simulink model "model_discrete"  (R2021b)
settings: Solver=FixedStepAuto  StartTime=0.0  StopTime=StopTime  FixedStep=T  RelTol=1e-3  EnableMultiTasking=on
undefined symbols (not defined in the file): K_disc, Knorm_disc, mtrxA_disc, mtrxB_disc, mtrxC_disc, Out, T
settings Model: Creator=vkad  LastModifiedBy=vkad
settings DataIOCC: ReturnWorkspaceOutputs=off
settings ModelReferenceCC: PropagateSignalLabelsOutOfModel=off

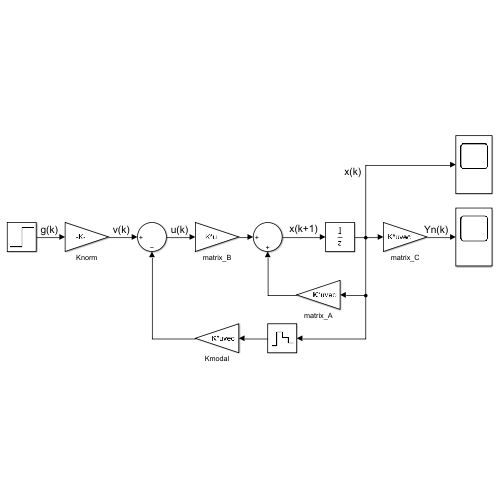
[thumbnail: Simulink's stored preview of the top-level diagram]
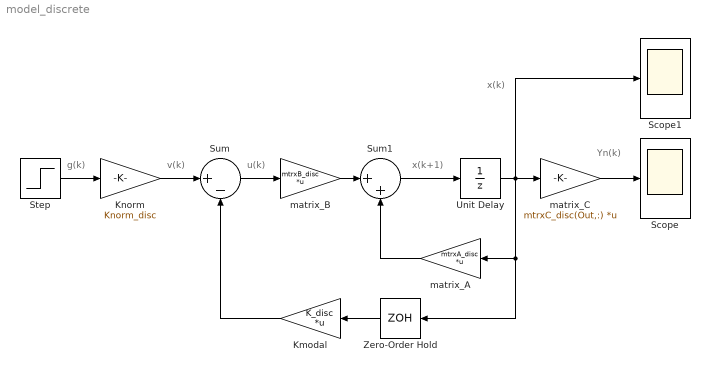
== system model_discrete ==
  note: v(k)
  note: u(k)
  note: x(k+1)
  note: x(k)
  note: Yn(k)
  note: g(k)
  Kmodal : Gain  Gain=K_disc  Multiplication=Matrix(K*u) (u vector)
  Knorm : Gain  Gain=Knorm_disc
  Scope : Scope
  Scope1 : Scope
  Step : Step  Time=0  SampleTime=0
  Sum : Sum  Inputs=|+-
  Sum1 : Sum  Inputs=|++
  Unit Delay : UnitDelay  SampleTime=T  HasFrameUpgradeWarning=on
  Zero-Order Hold : ZeroOrderHold  SampleTime=T
  matrix_A : Gain  Gain=mtrxA_disc  Multiplication=Matrix(K*u) (u vector)
  matrix_B : Gain  Gain=mtrxB_disc  Multiplication=Matrix(K*u)
  matrix_C : Gain  Gain=mtrxC_disc(Out,:)  Multiplication=Matrix(K*u) (u vector)
  wires:
  Step/1 -> Knorm/1
  Knorm/1 -> Sum/1
  Sum/1 -> matrix_B/1
  matrix_B/1 -> Sum1/1
  Sum1/1 -> Unit Delay/1
  Unit Delay/1 -> matrix_A/1, Zero-Order Hold/1, matrix_C/1, Scope1/1
  matrix_A/1 -> Sum1/2
  Zero-Order Hold/1 -> Kmodal/1
  Kmodal/1 -> Sum/2
  matrix_C/1 -> Scope/1
